simulink model "Lab0_ECE_ME_360_2019a"  (R2020b)
settings: Solver=ode1  StartTime=0.0  StopTime=inf  FixedStep=0.001  RelTol=1e-3
values from neighbouring files (symbols this model uses):
  Kt = 0.00767    [Inverted_Pendulum9_data.m]
  Nenc = 4096    [Inverted_Pendulum9_data.m]
  R = 2.6    [Inverted_Pendulum9_data.m]
  rg = 3.71    [Inverted_Pendulum9_data.m]
  rm = 6.35e-3    (= 0.00635)    [Inverted_Pendulum9_data.m]
  T = 0.001    [Inverted_Pendulum9_data.m]
  Vmax = 5    [Inverted_Pendulum9_data.m]
undefined symbols (not defined in the file or in its folder): binb1, binb2, binb3, binW1, binW2, binW3, control1b1, control1b2, control1b3, control1W1, control1W2, control1W3, control2b1, control2b2, control2b3, control2W1, control2W2, control2W3, control3b1, control3b2, control3b3, control3W1, control3W2, control3W3, HIL, qc_get_step_size, r_enc
libraries: quarc_library x7
settings Model: SimulationMode=external  ExtModeTrigDuration=5000  Creator=johnchiasson  LastModifiedBy=nardosashenafi
settings SolverCC: PositivePriorityOrder=on
settings DataIOCC: LimitDataPoints=on  SaveFormat=Array  ReturnWorkspaceOutputs=off
settings OptimizationCC: LifeSpan=inf
settings DebuggingCC: SFUnexpectedBacktrackingDiag=warning  SFNoUnconditionalDefaultTransitionDiag=warning  SFExecutionAtInitializationDiag=none  ArithmeticOperatorsInVariantConditions=warning
settings HardwareCC: ProdBitPerPointer=32  ProdBitPerSizeT=32  ProdBitPerPtrDiffT=32  ProdLargestAtomicFloat=None  ProdIntDivRoundTo=Undefined  ProdEndianess=Unspecified  ProdWordSize=32  ProdHWDeviceType=32-bit Generic
settings ModelReferenceCC: PropagateSignalLabelsOutOfModel=off
settings SFSimCC: SimUseLocalCustomCode=off  CustomCodeUndefinedFunction=UseInterfaceOnly
settings RTWCC: Description=QUARC Win64 Target  SystemTargetFile=quarc_win64.tlc  TemplateMakefile=quarc_default_tmf  RTWUseLocalCustomCode=off
settings CodeAppCC: StateflowObjectComments=on
settings STFCustomTargetCC: TargetPreCompLibLocation=C:\PROGRA~3\QUARC\lib\2019a\win64\release  CPPClassGenCompliant=off
settings GRTTargetCC: TargetPreCompLibLocation=C:\PROGRA~3\QUARC\lib\2019a\win64\release  TargetLangStandard=C89/C90 (ANSI)  ParMdlRefBuildCompliant=off  CompOptLevelCompliant=off  CombineOutputUpdateFcns=off  MatFileLogging=off  CPPClassGenCompliant=off  GRTInterface=on  UseToolchainInfoCompliant=off  ExtMode=on  ExtModeMexFile=quarc_comm
settings ConfigComp: CovMetricSettings=dw  CovSaveCumulativeToWorkspaceVar=on  CovSaveSingleToWorkspaceVar=on  CovExternalEMLEnable=off

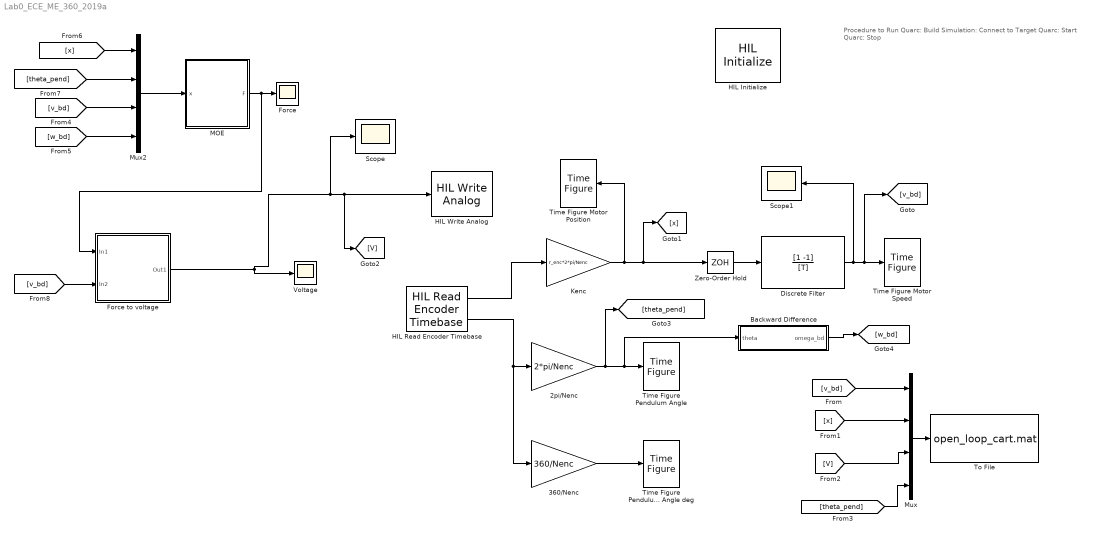
== system Lab0_ECE_ME_360_2019a ==
  note: Procedure to Run
      |
      | Quarc: Build
      | Simulation: Connect to Target
      | Quarc: Start
      | Quarc: Stop
  2pi/Nenc : Gain  Gain=2*pi/Nenc
  360/Nenc : Gain  Gain=360/Nenc
  Backward Difference : Subsystem
  Discrete Filter : DiscreteFilter  Numerator=[1 -1]  Denominator=[T]
  Force : Scope
  Force to voltage : Subsystem
  HIL Initialize : quarc_library/Data Acquisition/Generic/Configuration/HIL Initialize  Priority=-99  object_name=HIL-1  board_type=q2_usb  board_number=0  board_options=d0=digital;d1=digital;led=auto;update_rate=normal;decimation=1  exclusive=off  active=off  hardware_clocks=[0]  clock_modes=[]  initial_clock_frequencies=[]  set_clock_params_at_start=off  set_clock_params_at_switch_in=off  set_clock_frequencies_at_start=off  set_clock_frequencies_at_switch_in=off  analog_input_channels=[0:1]  analog_input_configurations=[]  analog_input_maximums=10  analog_input_minimums=-10  set_analog_input_params_at_start=on  set_analog_input_params_at_switch_in=off  analog_output_channels=[0:1]  analog_output_maximums=10  analog_output_minimums=-10  initial_analog_outputs=[0]  final_analog_outputs=[0]  watchdog_analog_outputs=0  set_analog_output_params_at_start=on  set_analog_output_params_at_switch_in=off  set_analog_outputs_at_start=on  set_analog_outputs_at_switch_in=off  set_analog_outputs_at_terminate=on  set_analog_outputs_at_switch_out=off  set_analog_outputs_on_watchdog=off  digital_input_channels=[]  digital_output_channels=[]  digital_output_configuration=[]  initial_digital_outputs=[1]  final_digital_outputs=[1]  watchdog_digital_outputs=[1]  set_digital_output_params_at_start=off  set_digital_output_params_at_switch_in=off  set_digital_outputs_at_start=on  set_digital_outputs_at_switch_in=off  set_digital_outputs_at_terminate=on  set_digital_outputs_at_switch_out=off  set_digital_outputs_on_watchdog=off  encoder_channels=[0:1]  quadrature=[4]  encoder_filter_frequency=[]  initial_encoder_counts=[0]  set_encoder_params_at_start=on  set_encoder_params_at_switch_in=off  set_encoder_counts_at_start=on  set_encoder_counts_at_switch_in=off  pwm_channels=[]  pwm_modes=[0]  pwm_frequency=1/0.020  pwm_configuration=[]  pwm_alignment=[]  pwm_polarity=[]  pwm_leading_deadband=[]  pwm_trailing_deadband=[]  initial_pwm_outputs=[0]  final_pwm_outputs=[0]  watchdog_pwm_outputs=[0]  set_pwm_params_at_start=on  set_pwm_params_at_switch_in=off  set_pwm_outputs_at_start=on  set_pwm_outputs_at_switch_in=off  set_pwm_outputs_at_terminate=on  set_pwm_outputs_at_switch_out=off  set_pwm_outputs_on_watchdog=off  other_output_channels=[]  initial_other_outputs=[]  final_other_outputs=[]  watchdog_other_outputs=[]  set_other_outputs_at_start=off  set_other_outputs_at_switch_in=off  set_other_outputs_at_terminate=off  set_other_outputs_at_switch_out=off  set_other_outputs_on_watchdog=off
  HIL Read Encoder Timebase : quarc_library/Data Acquisition/Generic/Timebases/HIL Read Encoder Timebase  object_name=HIL-1  clock=0  channels=[0:1]  samples_in_buffer=max(ceil(1/qc_get_step_size), 1)  active=on  vector_output=off  data_type_mode=Inherit via back propagation  data_type=double
  HIL Write Analog : quarc_library/Data Acquisition/Generic/Immediate I//O/HIL Write Analog  object_name=HIL-1  channels=0  sample_time=-1  active=off  vector_input=off
  Kenc : Gain  Gain=r_enc*2*pi/Nenc
  MOE : Subsystem
  Mux : Mux
  Mux2 : Mux
  Scope : Scope
  Scope1 : Scope
  Time Figure Motor Position : quarc_library/Sinks/Figures/Time Figure  figure_mode=Use figure window  figure_tag=figure1  axes_tag=axes1  minimum_y=-1  maximum_y=1  buffer_size=10000  update_rate=10  initial_position="440  227  720  450"  initial_visibility=off  sample_time=-1  relative_time=off
      settings: SourceProductName=QUARC Targets
  Time Figure Motor Speed : quarc_library/Sinks/Figures/Time Figure  figure_mode=Use figure window  figure_tag=figure1  axes_tag=axes1  minimum_y=-1  maximum_y=1  buffer_size=10000  update_rate=10  initial_position="440  227  720  450"  initial_visibility=off  sample_time=-1  relative_time=off
      settings: SourceProductName=QUARC Targets
  Time Figure Pendulum Angle : quarc_library/Sinks/Figures/Time Figure  figure_mode=Use figure window  figure_tag=figure1  axes_tag=axes1  minimum_y=-1  maximum_y=1  buffer_size=10000  update_rate=10  initial_position="5   33  712  818"  initial_visibility=off  sample_time=-1  relative_time=off
      settings: SourceProductName=QUARC Targets
  Time Figure Pendulum Angle deg : quarc_library/Sinks/Figures/Time Figure  figure_mode=Use figure window  figure_tag=figure1  axes_tag=axes1  minimum_y=-1  maximum_y=1  buffer_size=10000  update_rate=10  initial_position="519  251  720  450"  initial_visibility=off  sample_time=-1  relative_time=off
      settings: SourceProductName=QUARC Targets
  To File : ToFile  Filename=open_loop_cart.mat  MatrixName=cart_data  SampleTime=T
  Voltage : Scope
  Zero-Order Hold : ZeroOrderHold  SampleTime=T
  wires:
  HIL Read Encoder Timebase/1 -> Kenc/1
  HIL Read Encoder Timebase/2 -> 360/Nenc/1, 2pi/Nenc/1
  Kenc/1 -> Time Figure Motor Position/1, [x], Zero-Order Hold/1
  2pi/Nenc/1 -> [theta_pend], Backward Difference/1(theta), Time Figure Pendulum Angle/1
  360/Nenc/1 -> Time Figure Pendulum Angle deg/1
  Zero-Order Hold/1 -> Discrete Filter/1
  Discrete Filter/1 -> Scope1/1, [v_bd], Time Figure Motor Speed/1
  Mux/1 -> To File/1
  [v_bd] -> Mux/1
  [x] -> Mux/2
  [V] -> Mux/3
  [theta_pend] -> Mux/4
  Force to voltage/1(Out1) -> HIL Write Analog/1, [V], Scope/1, Voltage/1
  [x] -> Mux2/1
  [v_bd] -> Mux2/3
  Mux2/1 -> MOE/1(x)
  [theta_pend] -> Mux2/2
  [v_bd] -> Force to voltage/2(In2)
  [w_bd] -> Mux2/4
  MOE/1(F) -> Force to voltage/1(In1), Force/1
  Backward Difference/1(omega_bd) -> [w_bd]

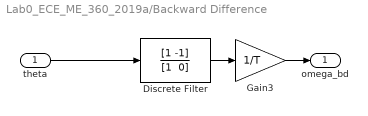
== system Lab0_ECE_ME_360_2019a/Backward Difference ==
  theta : Inport
  Discrete Filter : DiscreteFilter  Numerator=[1 -1]  Denominator="[1  0]"
  Gain3 : Gain  Gain=1/T  SaturateOnIntegerOverflow=on  OutDataTypeStr=Inherit: Same as input  ParamDataTypeStr=Inherit: Same as input
  omega_bd : Outport  VectorParamsAs1DForOutWhenUnconnected=off
  wires:
  Discrete Filter/1 -> Gain3/1
  Gain3/1 -> omega_bd/1
  theta/1 -> Discrete Filter/1

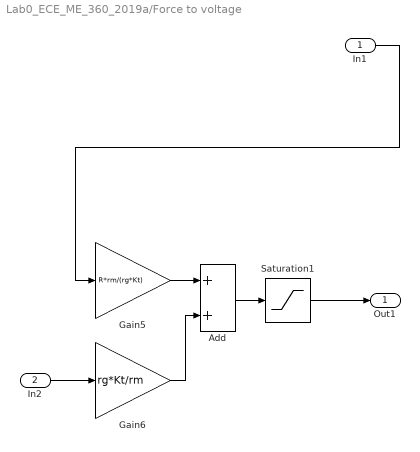
== system Lab0_ECE_ME_360_2019a/Force to voltage ==
  In1 : Inport
  In2 : Inport  Port=2
  Add : Sum
  Gain5 : Gain  Gain=R*rm/(rg*Kt)  SaturateOnIntegerOverflow=on  OutDataTypeStr=Inherit: Same as input  ParamDataTypeStr=Inherit: Same as input
  Gain6 : Gain  Gain=rg*Kt/rm  SaturateOnIntegerOverflow=on  OutDataTypeStr=Inherit: Same as input  ParamDataTypeStr=Inherit: Same as input
  Saturation1 : Saturate  UpperLimit=Vmax  LowerLimit=-Vmax
  Out1 : Outport
  wires:
  Add/1 -> Saturation1/1
  Gain5/1 -> Add/1
  Saturation1/1 -> Out1/1
  In1/1 -> Gain5/1
  Gain6/1 -> Add/2
  In2/1 -> Gain6/1

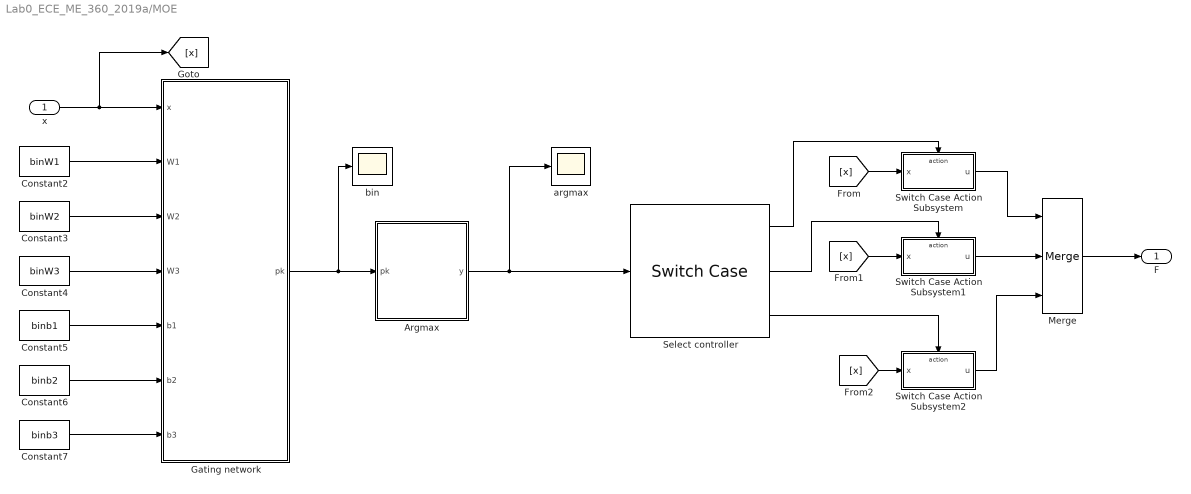
== system Lab0_ECE_ME_360_2019a/MOE ==
  x : Inport
  Argmax : MATLAB Function  TreatAsAtomicUnit=on
  Constant2 : Constant  Value=binW1
  Constant3 : Constant  Value=binW2
  Constant4 : Constant  Value=binW3
  Constant5 : Constant  Value=binb1
  Constant6 : Constant  Value=binb2
  Constant7 : Constant  Value=binb3
  Gating network : MATLAB Function  TreatAsAtomicUnit=on
  Merge : Merge  Inputs=3
  Select controller : SwitchCase  CaseConditions={1, 2, 3}  ShowDefaultCase=off
  Switch Case Action Subsystem : Subsystem  TreatAsAtomicUnit=on
  Switch Case Action Subsystem1 : Subsystem  TreatAsAtomicUnit=on
  Switch Case Action Subsystem2 : Subsystem  TreatAsAtomicUnit=on
  argmax : Scope
  bin : Scope
  F : Outport  VectorParamsAs1DForOutWhenUnconnected=off
  wires:
  Constant3/1 -> Gating network/3(W2)
  Constant7/1 -> Gating network/7(b3)
  Constant5/1 -> Gating network/5(b1)
  Constant4/1 -> Gating network/4(W3)
  Constant6/1 -> Gating network/6(b2)
  Gating network/1(pk) -> Argmax/1(pk), bin/1
  Constant2/1 -> Gating network/2(W1)
  x/1 -> [x], Gating network/1(x)
  Argmax/1(y) -> argmax/1, Select controller/1
  Select controller/1 -> Switch Case Action Subsystem/Action
  Select controller/2 -> Switch Case Action Subsystem1/Action
  Select controller/3 -> Switch Case Action Subsystem2/Action
  [x] -> Switch Case Action Subsystem2/1(x)
  [x] -> Switch Case Action Subsystem1/1(x)
  [x] -> Switch Case Action Subsystem/1(x)
  Switch Case Action Subsystem/1(u) -> Merge/1
  Switch Case Action Subsystem1/1(u) -> Merge/2
  Switch Case Action Subsystem2/1(u) -> Merge/3
  Merge/1 -> F/1

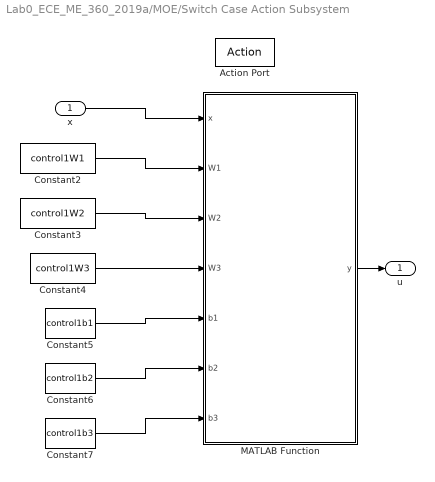
== system Lab0_ECE_ME_360_2019a/MOE/Switch Case Action Subsystem ==
  x : Inport
  Action Port : ActionPort
  Constant2 : Constant  Value=control1W1
  Constant3 : Constant  Value=control1W2
  Constant4 : Constant  Value=control1W3  VectorParams1D=off
  Constant5 : Constant  Value=control1b1
  Constant6 : Constant  Value=control1b2
  Constant7 : Constant  Value=control1b3
  MATLAB Function : MATLAB Function  TreatAsAtomicUnit=on
  u : Outport
  wires:
  Constant2/1 -> MATLAB Function/2(W1)
  Constant5/1 -> MATLAB Function/5(b1)
  Constant7/1 -> MATLAB Function/7(b3)
  Constant6/1 -> MATLAB Function/6(b2)
  Constant4/1 -> MATLAB Function/4(W3)
  Constant3/1 -> MATLAB Function/3(W2)
  x/1 -> MATLAB Function/1(x)
  MATLAB Function/1(y) -> u/1

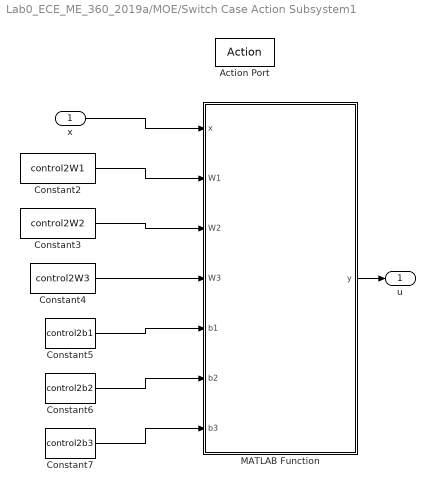
== system Lab0_ECE_ME_360_2019a/MOE/Switch Case Action Subsystem1 ==
  x : Inport
  Action Port : ActionPort
  Constant2 : Constant  Value=control2W1
  Constant3 : Constant  Value=control2W2
  Constant4 : Constant  Value=control2W3  VectorParams1D=off
  Constant5 : Constant  Value=control2b1
  Constant6 : Constant  Value=control2b2
  Constant7 : Constant  Value=control2b3
  MATLAB Function : MATLAB Function  TreatAsAtomicUnit=on
  u : Outport
  wires:
  Constant7/1 -> MATLAB Function/7(b3)
  Constant2/1 -> MATLAB Function/2(W1)
  Constant3/1 -> MATLAB Function/3(W2)
  Constant4/1 -> MATLAB Function/4(W3)
  MATLAB Function/1(y) -> u/1
  x/1 -> MATLAB Function/1(x)
  Constant6/1 -> MATLAB Function/6(b2)
  Constant5/1 -> MATLAB Function/5(b1)

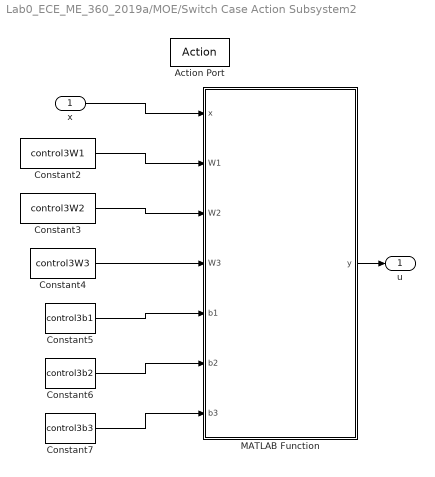
== system Lab0_ECE_ME_360_2019a/MOE/Switch Case Action Subsystem2 ==
  x : Inport
  Action Port : ActionPort
  Constant2 : Constant  Value=control3W1
  Constant3 : Constant  Value=control3W2
  Constant4 : Constant  Value=control3W3  VectorParams1D=off
  Constant5 : Constant  Value=control3b1
  Constant6 : Constant  Value=control3b2
  Constant7 : Constant  Value=control3b3
  MATLAB Function : MATLAB Function  TreatAsAtomicUnit=on
  u : Outport
  wires:
  Constant7/1 -> MATLAB Function/7(b3)
  Constant2/1 -> MATLAB Function/2(W1)
  Constant3/1 -> MATLAB Function/3(W2)
  Constant4/1 -> MATLAB Function/4(W3)
  MATLAB Function/1(y) -> u/1
  x/1 -> MATLAB Function/1(x)
  Constant6/1 -> MATLAB Function/6(b2)
  Constant5/1 -> MATLAB Function/5(b1)

== matlab function Lab0_ECE_ME_360_2019a/MOE/Argmax ==
  data: pk input; y output
function y = fcn(pk)
    maxindex = 1;
    for i = 1:length(pk)-1
       if pk(i+1) > pk(maxindex)
           maxindex = i+1;
       end
    end
y = maxindex;

== matlab function Lab0_ECE_ME_360_2019a/MOE/Gating network ==
  data: x input; W1 input; pk output; W2 input; W3 input; b1 input; b2 input; b3 input
function pk = fcn(x, W1, W2, W3, b1, b2, b3)

    z0 = [x(1); cos(x(2)); sin(x(2)); x(3); x(4)];
    z1 = elu(W1*z0 + b1);
    z2 = elu(W2*z1 + b2);
    z3 = elu(W3*z2 + b3);
    pk = softmax(z3);
    
end
    
function y = softmax(x)
    y = zeros(length(x));
    for i =1:length(x)
        y(i) = exp(x(i))/sum(exp(x));
    end
end

== matlab function Lab0_ECE_ME_360_2019a/MOE/Switch Case Action Subsystem/MATLAB Function ==
  data: x input; y output; W1 input; W2 input; W3 input; b1 input; b2 input; b3 input
function y = fcn(x, W1, W2, W3, b1, b2, b3)
    z0 = [x(1); cos(x(2)); sin(x(2)); x(3); x(4)];
    z1 = elu(W1*z0 + b1);
    z2 = elu(W2*z1 + b2);
    z3 = elu(W3*z2 + b3);
y = z3;

== matlab function Lab0_ECE_ME_360_2019a/MOE/Switch Case Action Subsystem1/MATLAB Function ==
  data: x input; y output; W1 input; W2 input; W3 input; b1 input; b2 input; b3 input
function y = fcn(x, W1, W2, W3, b1, b2, b3)
    z0 = [x(1); cos(x(2)); sin(x(2)); x(3); x(4)];
    z1 = elu(W1*z0 + b1);
    z2 = elu(W2*z1 + b2);
    z3 = elu(W3*z2 + b3);
y = z3;

== matlab function Lab0_ECE_ME_360_2019a/MOE/Switch Case Action Subsystem2/MATLAB Function ==
  data: x input; y output; W1 input; W2 input; W3 input; b1 input; b2 input; b3 input
function y = fcn(x, W1, W2, W3, b1, b2, b3)
    z0 = [x(1); cos(x(2)); sin(x(2)); x(3); x(4)];
    z1 = elu(W1*z0 + b1);
    z2 = elu(W2*z1 + b2);
    z3 = elu(W3*z2 + b3);
y = z3;
